simulink model "lab3model"  (R2021a)
settings: Solver=VariableStepAuto  StartTime=0.0  StopTime=40  RelTol=1e-3
values from neighbouring files (symbols this model uses):
  K2 = 0.0609    [lab3_sim.m]
  K3 = -4.419    [lab3_sim.m]
settings Model: Creator=ajendo  LastModifiedBy=adrian

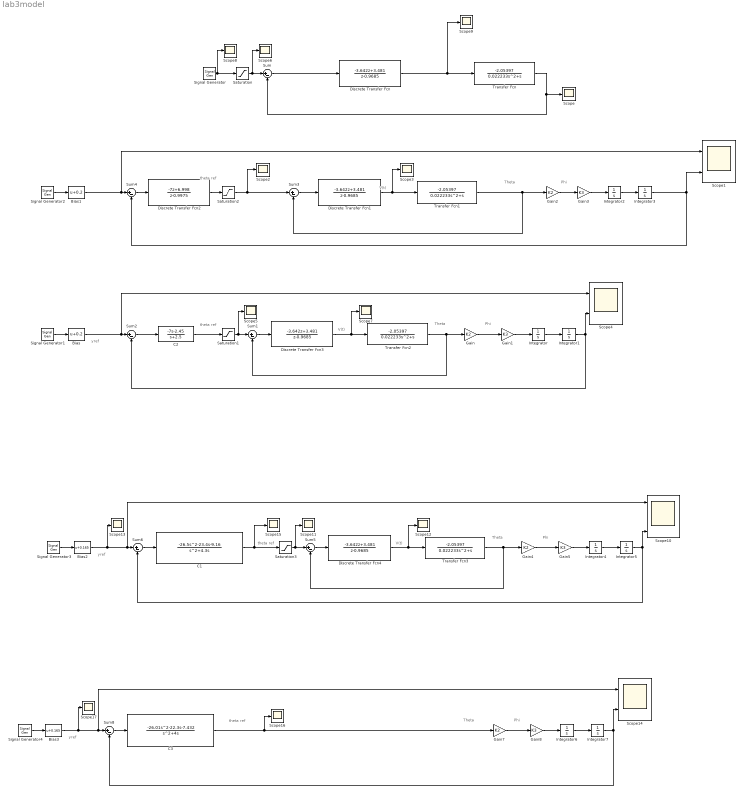
== system lab3model ==
  note: theta ref
  note: yref
  note: Phi
  note: Theta
  note: V(t)
  note: theta ref
  note: Phi
  note: Theta
  note: V(t)
  note: Phi
  note: yref
  note: Theta
  note: V(t)
  note: theta ref
  note: Theta
  note: theta ref
  note: yref
  note: Phi
  Bias : Bias  Bias=0.2
  Bias1 : Bias  Bias=0.2
  Bias2 : Bias  Bias=0.165
  Bias3 : Bias  Bias=0.165
  C1 : TransferFcn  Numerator=[-26.5 -23.4 -9.16]  Denominator=[1 4.3 0]
  C2 : TransferFcn  Numerator=[-7 -2.45]  Denominator=[1 2.5]
  C3 : TransferFcn  Numerator=[-26.01 -22.3 -7.432]  Denominator=[1 4 0]
  Discrete Transfer Fcn{,1,3..4} (4 alike) : DiscreteTransferFcn  Numerator=[-3.642 3.481]  Denominator=[1 -0.9685]  SampleTime=[0.001, 0]
  Discrete Transfer Fcn2 : DiscreteTransferFcn  Numerator=[-7 6.998]  Denominator=[1 -0.9975]  SampleTime=[0.001, 0]
  Gain{,2,4,7} (4 alike) : Gain  Gain=K2
  Gain{1,3,5,8} (4 alike) : Gain  Gain=K3
  Integrator{,1..7} (8 alike) : Integrator
  Saturation{,1..3} (4 alike) : Saturate  UpperLimit=0.7  LowerLimit=-0.7
  Scope{,2..3,5..9,11..13,15..17} (14 alike) : Scope
  Scope1 : Scope  NumInputPorts=2
  Scope10 : Scope  NumInputPorts=3
  Scope14 : Scope  NumInputPorts=2
  Scope4 : Scope  NumInputPorts=2
  Signal Generator : SignalGenerator  WaveForm=square  Amplitude=2  Units=rad/sec
  Signal Generator1 : SignalGenerator  WaveForm=square  Amplitude=0.05  Frequency=0.05
  Signal Generator2 : SignalGenerator  WaveForm=square  Amplitude=0.05  Frequency=0.05
  Signal Generator3 : SignalGenerator  WaveForm=square  Amplitude=0.015  Frequency=0.025
  Signal Generator4 : SignalGenerator  WaveForm=square  Amplitude=0.015  Frequency=0.025
  Sum{,1..6,8} (8 alike) : Sum  Inputs=|+-
  Transfer Fcn{,1..3} (4 alike) : TransferFcn  Numerator=[-2.05397]  Denominator=[0.022233 1 0]
  wires:
  Transfer Fcn2/1 -> Gain/1, Sum1/2
  Saturation1/1 -> Scope5/1, Sum1/1
  Signal Generator1/1 -> Bias/1
  Bias/1 -> Scope4/1, Sum2/1
  Gain/1 -> Gain1/1
  Gain1/1 -> Integrator/1
  Integrator/1 -> Integrator1/1
  Discrete Transfer Fcn3/1 -> Transfer Fcn2/1, Scope7/1
  Sum1/1 -> Discrete Transfer Fcn3/1
  C2/1 -> Saturation1/1
  Integrator1/1 -> Scope4/2, Sum2/2
  Sum2/1 -> C2/1
  Signal Generator2/1 -> Bias1/1
  Discrete Transfer Fcn1/1 -> Transfer Fcn1/1, Scope3/1
  Gain3/1 -> Integrator2/1
  Integrator2/1 -> Integrator3/1
  Gain2/1 -> Gain3/1
  Bias1/1 -> Scope1/1, Sum4/1
  Discrete Transfer Fcn2/1 -> Saturation2/1
  Sum4/1 -> Discrete Transfer Fcn2/1
  Sum3/1 -> Discrete Transfer Fcn1/1
  Saturation2/1 -> Sum3/1, Scope2/1
  Integrator3/1 -> Sum4/2, Scope1/2
  Transfer Fcn1/1 -> Gain2/1, Sum3/2
  Discrete Transfer Fcn/1 -> Scope9/1, Transfer Fcn/1
  Sum/1 -> Discrete Transfer Fcn/1
  Transfer Fcn/1 -> Sum/2, Scope/1
  Signal Generator/1 -> Scope8/1, Saturation/1
  Saturation/1 -> Scope6/1, Sum/1
  Discrete Transfer Fcn4/1 -> Transfer Fcn3/1, Scope12/1
  Integrator4/1 -> Integrator5/1
  Gain4/1 -> Gain5/1
  Sum6/1 -> C1/1
  Sum5/1 -> Discrete Transfer Fcn4/1
  Gain5/1 -> Integrator4/1
  Integrator5/1 -> Scope10/3, Sum6/2
  Saturation3/1 -> Scope11/1, Sum5/1
  Signal Generator3/1 -> Bias2/1
  Bias2/1 -> Scope13/1, Scope10/1, Sum6/1
  Transfer Fcn3/1 -> Gain4/1, Sum5/2
  Bias3/1 -> Scope17/1, Scope14/1, Sum8/1
  Signal Generator4/1 -> Bias3/1
  Integrator7/1 -> Scope14/2, Sum8/2
  Sum8/1 -> C3/1
  Gain8/1 -> Integrator6/1
  Integrator6/1 -> Integrator7/1
  Gain7/1 -> Gain8/1
  C3/1 -> Scope16/1, Gain7/1
  C1/1 -> Saturation3/1, Scope15/1
